simulink model "ME419_Ex1_6"  (R2023b)
settings: Solver=VariableStepAuto  StartTime=0.0  StopTime=10.0  RelTol=1e-6
settings Model: Creator=aliawolken  LastModifiedBy=aliawolken

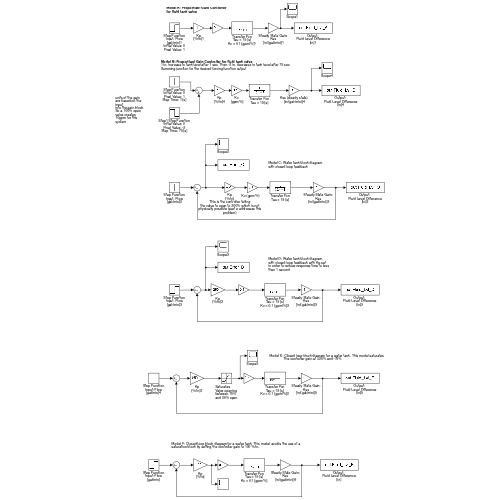
[thumbnail: Simulink's stored preview of the top-level diagram]
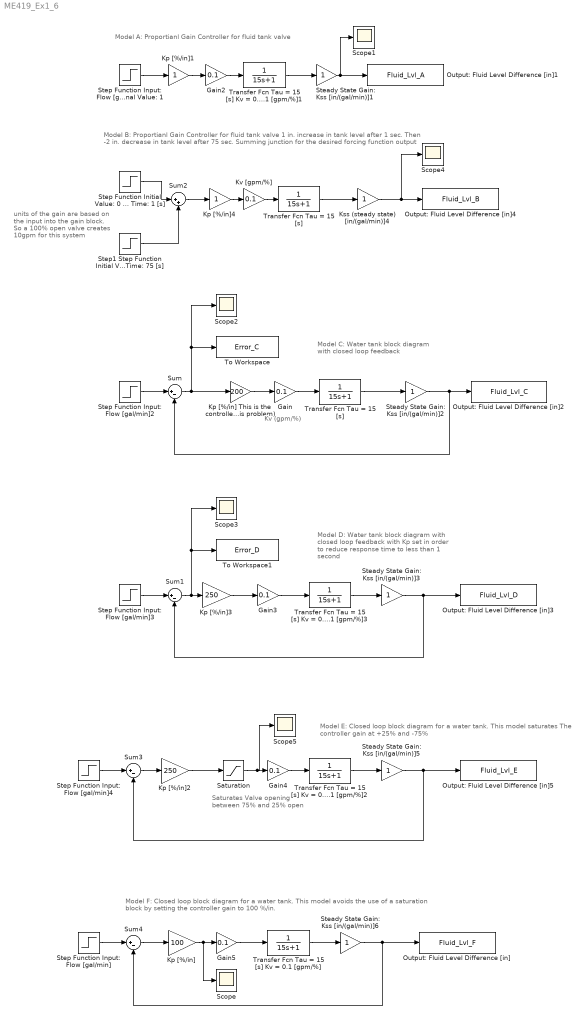
== system ME419_Ex1_6 ==
  note: units of the gain are based on the input
      | into the gain block. So a 100% open valve creates 10gpm for this system
  note: Model F: Closed loop block diagram for a water tank. This model avoids the use of a saturation block by setting the controller gain to 100 %/in.
  note: Model E: Closed loop block diagram for a water tank. This model saturates
      | 		The controller gain at +25% and -75%
  note: Model D: Water tank block diagram
      | with closed loop feedback with Kp set
      | in order to reduce response time to less
      | than 1 second
  note: Model C: Water tank block diagram
      | with closed loop feedback
  note: Model B: Proportianl Gain Controller for fluid tank valve
      | 1 in. increase in tank level after 1 sec. Then -2 in. decrease in tank level after 75 sec. Summing junction for the desired forcing function output
  note: Model A: Proportianl Gain Controller
      | for fluid tank valve
  note: Saturates
      | Valve opening
      | between 75%
      | and 25% open
  note: Kv (gpm/%)
  Gain{,2..5} (5 alike) : Gain  Gain=0.1
  Kp [%/in] : Gain  Gain=100
  "Kp [%/in] This is the controller telling the valve to open to 200% which is not physically possible (part e addresses this problem) " : Gain  Gain=200
  Kp [%/in]1 : Gain
  Kp [%/in]2 : Gain  Gain=250
  Kp [%/in]3 : Gain  Gain=250
  Kp [%/in]4 : Gain
  Kss (steady state) [in/(gal/min)]4 : Gain
  Kv [gpm/%] : Gain  Gain=0.1
  Output: Fluid Level Difference [in] : ToWorkspace  VariableName=Fluid_Lvl_F  SampleTime=-1
  Output: Fluid Level Difference [in]1 : ToWorkspace  VariableName=Fluid_Lvl_A  SampleTime=-1
  Output: Fluid Level Difference [in]2 : ToWorkspace  VariableName=Fluid_Lvl_C  SampleTime=-1
  Output: Fluid Level Difference [in]3 : ToWorkspace  VariableName=Fluid_Lvl_D  SampleTime=-1
  Output: Fluid Level Difference [in]4 : ToWorkspace  VariableName=Fluid_Lvl_B  SampleTime=-1
  Output: Fluid Level Difference [in]5 : ToWorkspace  VariableName=Fluid_Lvl_E  SampleTime=-1
  Saturation : Saturate  UpperLimit=25  LowerLimit=-75
  Scope{,1..5} (6 alike) : Scope
  Steady State Gain: Kss [in/(gal/min)]{1..3,5..6} (5 alike) : Gain
  Step Function Initial Value: 0 Final Value: 1 Step Time: 1 [s] : Step  SampleTime=0
  Step Function Input: Flow [gal/min]{,2..4} (4 alike) : Step  SampleTime=0
  Step Function Input: Flow [gal/min]1 Initial Value: 0 Final Value: 1 : Step  SampleTime=0
  Step1 Step Function Initial Value: 0 Final Value: -2 Step Time: 75 [s] : Step  Time=75  After=-2  SampleTime=0
  Sum{,1,3..4} (4 alike) : Sum  Inputs=|+-
  Sum2 : Sum  Inputs=|++
  To Workspace : ToWorkspace  VariableName=Error_C  SampleTime=-1
  To Workspace1 : ToWorkspace  VariableName=Error_D  SampleTime=-1
  Transfer Fcn Tau = 15 [s] : TransferFcn  Denominator=[15 1]
  "Transfer Fcn Tau = 15 [s] " : TransferFcn  Denominator=[15 1]
  Transfer Fcn Tau = 15 [s] Kv = 0.1 [gpm/%]{,1..3} (4 alike) : TransferFcn  Denominator=[15 1]
  wires:
  Steady State Gain: Kss [in/(gal/min)]1/1 -> Scope1/1, Output: Fluid Level Difference [in]1/1
  Transfer Fcn Tau = 15 [s] Kv = 0.1 [gpm/%]1/1 -> Steady State Gain: Kss [in/(gal/min)]1/1
  Kp [%/in]1/1 -> Gain2/1
  Step Function Input: Flow [gal/min]1 Initial Value: 0 Final Value: 1/1 -> Kp [%/in]1/1
  "Kp [%/in] This is the controller telling the valve to open to 200% which is not physically possible (part e addresses this problem) "/1 -> Gain/1
  Transfer Fcn Tau = 15 [s]/1 -> Steady State Gain: Kss [in/(gal/min)]2/1
  Step Function Input: Flow [gal/min]2/1 -> Sum/1
  Sum/1 -> Scope2/1, To Workspace/1, "Kp [%/in] This is the controller telling the valve to open to 200% which is not physically possible (part e addresses this problem) "/1
  Steady State Gain: Kss [in/(gal/min)]2/1 -> Sum/2, Output: Fluid Level Difference [in]2/1
  Steady State Gain: Kss [in/(gal/min)]3/1 -> Sum1/2, Output: Fluid Level Difference [in]3/1
  Transfer Fcn Tau = 15 [s] Kv = 0.1 [gpm/%]3/1 -> Steady State Gain: Kss [in/(gal/min)]3/1
  Kp [%/in]3/1 -> Gain3/1
  Step Function Input: Flow [gal/min]3/1 -> Sum1/1
  Sum1/1 -> Scope3/1, To Workspace1/1, Kp [%/in]3/1
  Step1 Step Function Initial Value: 0 Final Value: -2 Step Time: 75 [s]/1 -> Sum2/2
  Step Function Initial Value: 0 Final Value: 1 Step Time: 1 [s]/1 -> Sum2/1
  "Transfer Fcn Tau = 15 [s] "/1 -> Kss (steady state) [in/(gal/min)]4/1
  Kss (steady state) [in/(gal/min)]4/1 -> Scope4/1, Output: Fluid Level Difference [in]4/1
  Kp [%/in]4/1 -> Kv [gpm/%]/1
  Sum2/1 -> Kp [%/in]4/1
  Gain/1 -> Transfer Fcn Tau = 15 [s]/1
  Kv [gpm/%]/1 -> "Transfer Fcn Tau = 15 [s] "/1
  Gain2/1 -> Transfer Fcn Tau = 15 [s] Kv = 0.1 [gpm/%]1/1
  Gain3/1 -> Transfer Fcn Tau = 15 [s] Kv = 0.1 [gpm/%]3/1
  Transfer Fcn Tau = 15 [s] Kv = 0.1 [gpm/%]2/1 -> Steady State Gain: Kss [in/(gal/min)]5/1
  Step Function Input: Flow [gal/min]4/1 -> Sum3/1
  Steady State Gain: Kss [in/(gal/min)]5/1 -> Sum3/2, Output: Fluid Level Difference [in]5/1
  Sum3/1 -> Kp [%/in]2/1
  Kp [%/in]2/1 -> Saturation/1
  Gain4/1 -> Transfer Fcn Tau = 15 [s] Kv = 0.1 [gpm/%]2/1
  Saturation/1 -> Scope5/1, Gain4/1
  Transfer Fcn Tau = 15 [s] Kv = 0.1 [gpm/%]/1 -> Steady State Gain: Kss [in/(gal/min)]6/1
  Step Function Input: Flow [gal/min]/1 -> Sum4/1
  Steady State Gain: Kss [in/(gal/min)]6/1 -> Sum4/2, Output: Fluid Level Difference [in]/1
  Sum4/1 -> Kp [%/in]/1
  Kp [%/in]/1 -> Scope/1, Gain5/1
  Gain5/1 -> Transfer Fcn Tau = 15 [s] Kv = 0.1 [gpm/%]/1
